simulink model "example2sim"  (Simulink 5.0)
settings: Solver=ode45  StartTime=0.0  StopTime=Tstop  RelTol=1e-3
values from neighbouring files (symbols this model uses):
  Cexp = expcon(Cimp,range)    [doubleintexp.m]    (also in example2.m = expcon(Cimp,range,options); mexexample1.m; regsiso.m; regulator.m)
libraries: hyblib x1, cstblocks x1
settings Model: LastModifiedBy=Xbemporad  ExtModeTrigMode=oneshot  ExtModeArmWhenConnect=off  LimitDataPoints=off  BooleanDataType=off

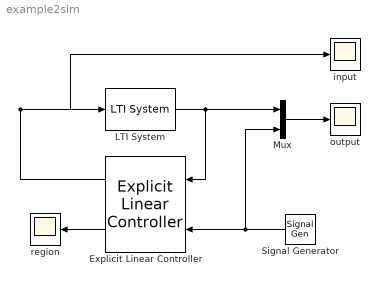
== system example2sim ==
  Explicit Linear Controller : hyblib/Explicit Linear Controller  Orientation=left  AncestorBlock=hyblib/Linear Constrained  C=Cexp  xhat0=[]  u1=[]  compile=on
  LTI System : cstblocks/LTI System  sys=tf(1,[1 2 1])  IC=[]
  Mux : Mux  Inputs=2
  Signal Generator : SignalGenerator  Orientation=left  WaveForm=sawtooth  Frequency=0.10
  input : Scope
      settings: TimeRange=20  YMin=-2  YMax=2
  output : Scope
      settings: TimeRange=20  YMin=-1  YMax=1
  region : Scope
      settings: TimeRange=10  YMin=0  YMax=10
  wires:
  Explicit Linear Controller/2 -> region/1
  LTI System/1 -> Mux/1, Explicit Linear Controller/1
  Mux/1 -> output/1
  Signal Generator/1 -> Mux/2, Explicit Linear Controller/2
  Explicit Linear Controller/1 -> LTI System/1, input/1
